simulink model "sim_tase_2025_pos_ctrl"  (R2020a)
settings: Solver=ode4  StartTime=0.0  StopTime=30.0  FixedStep=0.01  RelTol=1e-3
values from neighbouring files (symbols this model uses):
  alfa_theta_obs = 100    [init_tase_2025_pos_ctrl.m]
  Aps = -diag([5, 5, 5])    [init_tase_2025_pos_ctrl.m]
  delta_p_i_0 = zeros(3, NF)    [init_tase_2025_pos_ctrl.m]
  delta_v_i_0 = zeros(3, NF)    [init_tase_2025_pos_ctrl.m]
  dp_aa_t = 0.2 * ones(3, 5) + ( 1.0 - 0.2 ) * rand(3, 5)    [init_tase_2025_pos_ctrl.m]
  dp_ff_t = [ 0.4 * ones(1, 5) + ( 1.0 - 0.4 ) * rand(1, 5);                      0.4 * ones(1, 5) + ( 1.0 - 0.4 ) * rand(1, 5);                      0.2 * ones(1, 5) + ( 0.6 - 0.2 ) * rand(1, 5) ]    [init_tase_2025_pos_ctrl.m]
  dp_phi_t = ( - pi / 2 ) * ones(3, 5) + ( pi / 2 - ( - pi / 2 ) ) * rand(3, 5)    [init_tase_2025_pos_ctrl.m]
  etai_0 = zeros(3,5)    [init_tase_2025_pos_ctrl.m]
  k_rho_1 = 10    [init_tase_2025_pos_ctrl.m]
  k_rho_2 = 10    [init_tase_2025_pos_ctrl.m]
  kai_1_t = 0.02    [init_tase_2025_pos_ctrl.m]
  kai_3_t = 0.1    [init_tase_2025_pos_ctrl.m]
  kp = 20    [init_tase_2025_pos_ctrl.m]
  ksii_0 = zeros(3,5)    [init_tase_2025_pos_ctrl.m]
  kv = 20    [init_tase_2025_pos_ctrl.m]
  l1v = diag([20; 20; 20])    [init_tase_2025_pos_ctrl.m]
  l2v = diag([30; 30; 30])    [init_tase_2025_pos_ctrl.m]
  mass_i = zeros(1,NF)    [init_tase_2025_pos_ctrl.m]
  Mii = diag([1;0;0;0;1])    [init_tase_2025_pos_ctrl.m]
  Phi_inv = inv( Aps ) * ( exp( Aps * tTs ) - eye(3) )    [init_tase_2025_pos_ctrl.m]
  pos0 = zeros(3, 1)    [init_tase_2025_pos_ctrl.m]
  PZ0 = P0(3)    [init_tase_2025_pos_ctrl.m]
  PZ1 = 10    [init_tase_2025_pos_ctrl.m]
  Qci_init = repmat([1;0;0;0],1,NF)    [init_tase_2025_pos_ctrl.m]
  R0 = 4    [init_tase_2025_pos_ctrl.m]
  R1 = 8    [init_tase_2025_pos_ctrl.m]
  Rx2 = 10    [init_tase_2025_pos_ctrl.m]
  Ry2 = 6    [init_tase_2025_pos_ctrl.m]
  Rz2 = 4    [init_tase_2025_pos_ctrl.m]
  T0 = 0    [init_tase_2025_pos_ctrl.m]
  T1 = tseq1    (= 10)    [init_tase_2025_pos_ctrl.m]
  T12 = tseq1 + tseq12    (= 20)    [init_tase_2025_pos_ctrl.m]
  T2 = tseq1 + tseq12 + tseq2    (= 30)    [init_tase_2025_pos_ctrl.m]
  theta0 = ( 2 / 5 ) * pi    (= 1.25663706144)    [init_tase_2025_pos_ctrl.m]
  theta_1 = 0    [init_tase_2025_pos_ctrl.m]
  theta_2 = 1    [init_tase_2025_pos_ctrl.m]
  TTb = 2    [init_tase_2025_pos_ctrl.m]
  tTs = 0.1    [init_tase_2025_pos_ctrl.m]
  vel0 = zeros(3, 1)    [init_tase_2025_pos_ctrl.m]
  Wij = [0,0,1,0,0;              0,0,1,1,0;              1,0,0,0,1;              0,1,1,0,0;              0,0,1,0,0]    [init_tase_2025_pos_ctrl.m]
  wp = 10    [init_tase_2025_pos_ctrl.m]
  X1 = 8    [init_tase_2025_pos_ctrl.m]
  X2 = 2    [init_tase_2025_pos_ctrl.m]
  X3 = 3    [init_tase_2025_pos_ctrl.m]
  Y1 = 10    [init_tase_2025_pos_ctrl.m]
  Y2 = 2    [init_tase_2025_pos_ctrl.m]
  Y3 = 4    [init_tase_2025_pos_ctrl.m]
  Z1 = 4    [init_tase_2025_pos_ctrl.m]
  Z2 = -6    [init_tase_2025_pos_ctrl.m]
  Z3 = 2    [init_tase_2025_pos_ctrl.m]
undefined symbols (not defined in the file or in its folder): cal_frac_squ, p_gamma1_pos, p_gamma1_vel, p_gamma2_pos, p_gamma2_vel, p_gamma_diff_1, p_gamma_diff_2_2, q_gamma1_pos, q_gamma1_vel, q_gamma2_pos, q_gamma2_vel, q_gamma_diff_1, q_gamma_diff_2_2
(part 3 of 4)

== matlab function sim_tase_2025_pos_ctrl/combine leader position estimaters ==
  data: ksi_d_est_1 input; ksi_d_est_vec output; ksi_d_est_2 input; ksi_d_est_3 input; ksi_d_est_4 input; ksi_d_est_5 input
function ksi_d_est_vec  = fcn(ksi_d_est_1, ksi_d_est_2, ksi_d_est_3, ksi_d_est_4, ksi_d_est_5)
%%%% 合并领导者位置观测器输出结果
ksi_d_est_vec = [ksi_d_est_1(:), ksi_d_est_2(:), ksi_d_est_3(:), ksi_d_est_4(:), ksi_d_est_5(:)];

== matlab function sim_tase_2025_pos_ctrl/combine lumped follower observation error  ==
  data: ksi_est_err_tilt_1 input; ksi_est_err_tilt_2 input; ksi_est_err_tilt_3 input; ksi_est_err_tilt_4 input; ksi_est_err_tilt_5 input; ksi_est_err_tilt_vec output; eta_est_err_tilt_1 input; eta_est_err_tilt_vec output; eta_est_err_tilt_2 input; eta_est_err_tilt_3 input; eta_est_err_tilt_4 input; eta_est_err_tilt_5 input
function [ksi_est_err_tilt_vec, eta_est_err_tilt_vec]  = fcn(ksi_est_err_tilt_1, ksi_est_err_tilt_2, ksi_est_err_tilt_3, ksi_est_err_tilt_4, ksi_est_err_tilt_5, ...
                                                                                                        eta_est_err_tilt_1, eta_est_err_tilt_2, eta_est_err_tilt_3, eta_est_err_tilt_4, eta_est_err_tilt_5)
%%%% 合并领导者位置观测器输出结果
ksi_est_err_tilt_vec = [ksi_est_err_tilt_1, ksi_est_err_tilt_2, ksi_est_err_tilt_3, ksi_est_err_tilt_4, ksi_est_err_tilt_5];
eta_est_err_tilt_vec = [eta_est_err_tilt_1, eta_est_err_tilt_2, eta_est_err_tilt_3, eta_est_err_tilt_4, eta_est_err_tilt_5];

== matlab function sim_tase_2025_pos_ctrl/combine lumped follower position observation error ==
  data: theta_ksi_est_err_tilt_1_1 input; theta_ksi_est_err_tilt_1_2 input; theta_ksi_est_err_tilt_1_3 input; theta_ksi_est_err_tilt_1_4 input; theta_ksi_est_err_tilt_1_5 input; theta_ksi_est_err_tilt_1_vec output; theta_ksi_est_err_tilt_2_1 input; theta_ksi_est_err_tilt_2_vec output; theta_ksi_est_err_tilt_2_2 input; theta_ksi_est_err_tilt_2_3 input; theta_ksi_est_err_tilt_2_4 input; theta_ksi_est_err_tilt_2_5 input
function [theta_ksi_est_err_tilt_1_vec, theta_ksi_est_err_tilt_2_vec]  = fcn(theta_ksi_est_err_tilt_1_1, theta_ksi_est_err_tilt_1_2, theta_ksi_est_err_tilt_1_3, theta_ksi_est_err_tilt_1_4, theta_ksi_est_err_tilt_1_5, ...
                                                                                                                                    theta_ksi_est_err_tilt_2_1, theta_ksi_est_err_tilt_2_2, theta_ksi_est_err_tilt_2_3, theta_ksi_est_err_tilt_2_4, theta_ksi_est_err_tilt_2_5)
%%%% 合并领导者位置观测器输出结果
theta_ksi_est_err_tilt_1_vec = [theta_ksi_est_err_tilt_1_1(:), theta_ksi_est_err_tilt_1_2(:), theta_ksi_est_err_tilt_1_3(:), theta_ksi_est_err_tilt_1_4(:), theta_ksi_est_err_tilt_1_5(:)];
theta_ksi_est_err_tilt_2_vec = [theta_ksi_est_err_tilt_2_1(:), theta_ksi_est_err_tilt_2_2(:), theta_ksi_est_err_tilt_2_3(:), theta_ksi_est_err_tilt_2_4(:), theta_ksi_est_err_tilt_2_5(:)];

== matlab function sim_tase_2025_pos_ctrl/combine lumped follower velocity observation error ==
  data: theta_eta_est_err_tilt_1_1 input; theta_eta_est_err_tilt_1_2 input; theta_eta_est_err_tilt_1_3 input; theta_eta_est_err_tilt_1_4 input; theta_eta_est_err_tilt_1_5 input; theta_eta_est_err_tilt_1_vec output; theta_eta_est_err_tilt_2_1 input; theta_eta_est_err_tilt_2_vec output; theta_eta_est_err_tilt_2_2 input; theta_eta_est_err_tilt_2_3 input; theta_eta_est_err_tilt_2_4 input; theta_eta_est_err_tilt_2_5 input
function [theta_eta_est_err_tilt_1_vec, theta_eta_est_err_tilt_2_vec]  = fcn(theta_eta_est_err_tilt_1_1, theta_eta_est_err_tilt_1_2, theta_eta_est_err_tilt_1_3, theta_eta_est_err_tilt_1_4, theta_eta_est_err_tilt_1_5, ...
                                                                                                                                    theta_eta_est_err_tilt_2_1, theta_eta_est_err_tilt_2_2, theta_eta_est_err_tilt_2_3, theta_eta_est_err_tilt_2_4, theta_eta_est_err_tilt_2_5)
%%%% 合并领导者位置观测器输出结果
theta_eta_est_err_tilt_1_vec = [theta_eta_est_err_tilt_1_1(:), theta_eta_est_err_tilt_1_2(:), theta_eta_est_err_tilt_1_3(:), theta_eta_est_err_tilt_1_4(:), theta_eta_est_err_tilt_1_5(:)];
theta_eta_est_err_tilt_2_vec = [theta_eta_est_err_tilt_2_1(:), theta_eta_est_err_tilt_2_2(:), theta_eta_est_err_tilt_2_3(:), theta_eta_est_err_tilt_2_4(:), theta_eta_est_err_tilt_2_5(:)];

== matlab function sim_tase_2025_pos_ctrl/fixed-time distributed follower desire position observer agent 1 ==
  data: l1p input; d_ksi_d_est_1 output; l2p input; eta_d_est_vec input; theta_ksi_est_err_tilt_1_vec input; theta_ksi_est_err_tilt_2_vec input
function d_ksi_d_est_1 = fcn(l1p, l2p, eta_d_est_vec, theta_ksi_est_err_tilt_1_vec, theta_ksi_est_err_tilt_2_vec)
%%%% 固定时间跟随者期望位置分布式观测器
iiuav = 1;
d_ksi_d_est_1 = eta_d_est_vec(:,iiuav) - l1p * theta_ksi_est_err_tilt_1_vec(:,iiuav) - l2p * theta_ksi_est_err_tilt_2_vec(:,iiuav);

== matlab function sim_tase_2025_pos_ctrl/fixed-time distributed follower desire position observer agent 2 ==
  data: l1p input; d_ksi_d_est_2 output; l2p input; eta_d_est_vec input; theta_ksi_est_err_tilt_1_vec input; theta_ksi_est_err_tilt_2_vec input
function d_ksi_d_est_2 = fcn(l1p, l2p, eta_d_est_vec, theta_ksi_est_err_tilt_1_vec, theta_ksi_est_err_tilt_2_vec)
%%%% 固定时间跟随者期望位置分布式观测器
iiuav = 2;
d_ksi_d_est_2 = eta_d_est_vec(:,iiuav) - l1p * theta_ksi_est_err_tilt_1_vec(:,iiuav) - l2p * theta_ksi_est_err_tilt_2_vec(:,iiuav);

== matlab function sim_tase_2025_pos_ctrl/update vl_hat agent 2 ==
  data: Aps input; d_vl_hat_2 output; ui0 input; ui1 input; dp_hat_vec input; vli_tilt_vec input
function d_vl_hat_2 = fcn(Aps, ui0, ui1, dp_hat_vec, vli_tilt_vec)
%%%% 更新状态预测器
iiuav = 2;
g0 = 9.80663;
e3 = [0;0;1];
d_vl_hat_2 = -g0 * e3 + ui0(:,iiuav) + dp_hat_vec(:,iiuav) ...
                        + ui1(:,iiuav) + Aps * vli_tilt_vec(:,iiuav);

== matlab function sim_tase_2025_pos_ctrl/fixed-time distributed follower desire position observer agent 3 ==
  data: l1p input; d_ksi_d_est_3 output; l2p input; eta_d_est_vec input; theta_ksi_est_err_tilt_1_vec input; theta_ksi_est_err_tilt_2_vec input
function d_ksi_d_est_3 = fcn(l1p, l2p, eta_d_est_vec, theta_ksi_est_err_tilt_1_vec, theta_ksi_est_err_tilt_2_vec)
%%%% 固定时间跟随者期望位置分布式观测器
iiuav = 3;
d_ksi_d_est_3 = eta_d_est_vec(:,iiuav) - l1p * theta_ksi_est_err_tilt_1_vec(:,iiuav) - l2p * theta_ksi_est_err_tilt_2_vec(:,iiuav);

== matlab function sim_tase_2025_pos_ctrl/fixed-time distributed follower desire position observer agent 4 ==
  data: l1p input; d_ksi_d_est_4 output; l2p input; eta_d_est_vec input; theta_ksi_est_err_tilt_1_vec input; theta_ksi_est_err_tilt_2_vec input
function d_ksi_d_est_4 = fcn(l1p, l2p, eta_d_est_vec, theta_ksi_est_err_tilt_1_vec, theta_ksi_est_err_tilt_2_vec)
%%%% 固定时间跟随者期望位置分布式观测器
iiuav = 4;
d_ksi_d_est_4 = eta_d_est_vec(:,iiuav) - l1p * theta_ksi_est_err_tilt_1_vec(:,iiuav) - l2p * theta_ksi_est_err_tilt_2_vec(:,iiuav);

== matlab function sim_tase_2025_pos_ctrl/fixed-time distributed follower desire position observer agent 5 ==
  data: l1p input; d_ksi_d_est_5 output; l2p input; eta_d_est_vec input; theta_ksi_est_err_tilt_1_vec input; theta_ksi_est_err_tilt_2_vec input
function d_ksi_d_est_5 = fcn(l1p, l2p, eta_d_est_vec, theta_ksi_est_err_tilt_1_vec, theta_ksi_est_err_tilt_2_vec)
%%%% 固定时间跟随者期望位置分布式观测器
iiuav = 5;
d_ksi_d_est_5 = eta_d_est_vec(:,iiuav) - l1p * theta_ksi_est_err_tilt_1_vec(:,iiuav) - l2p * theta_ksi_est_err_tilt_2_vec(:,iiuav);

== matlab function sim_tase_2025_pos_ctrl/fixed-time distributed follower desire velocity observer agent 1 ==
  data: l1v input; d_eta_d_est_1 output; l2v input; theta_eta_est_err_tilt_1_vec input; theta_eta_est_err_tilt_2_vec input
function d_eta_d_est_1 = fcn(l1v, l2v, theta_eta_est_err_tilt_1_vec, theta_eta_est_err_tilt_2_vec)
%%%% 固定时间跟随者期望速度分布式观测器
iiuav = 1;
d_eta_d_est_1 = -l1v * theta_eta_est_err_tilt_1_vec(:,iiuav) - l2v * theta_eta_est_err_tilt_2_vec(:,iiuav);

== matlab function sim_tase_2025_pos_ctrl/fixed-time distributed follower desire velocity observer agent 2 ==
  data: l1v input; d_eta_d_est_2 output; l2v input; theta_eta_est_err_tilt_1_vec input; theta_eta_est_err_tilt_2_vec input
function d_eta_d_est_2 = fcn(l1v, l2v, theta_eta_est_err_tilt_1_vec, theta_eta_est_err_tilt_2_vec)
%%%% 固定时间跟随者期望速度分布式观测器
iiuav = 2;
d_eta_d_est_2 = -l1v * theta_eta_est_err_tilt_1_vec(:,iiuav) - l2v * theta_eta_est_err_tilt_2_vec(:,iiuav);

== matlab function sim_tase_2025_pos_ctrl/fixed-time distributed follower desire velocity observer agent 3 ==
  data: l1v input; d_eta_d_est_3 output; l2v input; theta_eta_est_err_tilt_1_vec input; theta_eta_est_err_tilt_2_vec input
function d_eta_d_est_3 = fcn(l1v, l2v, theta_eta_est_err_tilt_1_vec, theta_eta_est_err_tilt_2_vec)
%%%% 固定时间跟随者期望速度分布式观测器
iiuav = 3;
d_eta_d_est_3 = -l1v * theta_eta_est_err_tilt_1_vec(:,iiuav) - l2v * theta_eta_est_err_tilt_2_vec(:,iiuav);

== matlab function sim_tase_2025_pos_ctrl/fixed-time distributed follower desire velocity observer agent 4 ==
  data: l1v input; d_eta_d_est_4 output; l2v input; theta_eta_est_err_tilt_1_vec input; theta_eta_est_err_tilt_2_vec input
function d_eta_d_est_4 = fcn(l1v, l2v, theta_eta_est_err_tilt_1_vec, theta_eta_est_err_tilt_2_vec)
%%%% 固定时间跟随者期望速度分布式观测器
iiuav = 4;
d_eta_d_est_4 = -l1v * theta_eta_est_err_tilt_1_vec(:,iiuav) - l2v * theta_eta_est_err_tilt_2_vec(:,iiuav);

== matlab function sim_tase_2025_pos_ctrl/fixed-time distributed follower desire velocity observer agent 5 ==
  data: l1v input; d_eta_d_est_5 output; l2v input; theta_eta_est_err_tilt_1_vec input; theta_eta_est_err_tilt_2_vec input
function d_eta_d_est_5 = fcn(l1v, l2v, theta_eta_est_err_tilt_1_vec, theta_eta_est_err_tilt_2_vec)
%%%% 固定时间跟随者期望速度分布式观测器
iiuav = 5;
d_eta_d_est_5 = -l1v * theta_eta_est_err_tilt_1_vec(:,iiuav) - l2v * theta_eta_est_err_tilt_2_vec(:,iiuav);

== matlab function sim_tase_2025_pos_ctrl/trans to column41 ==
  data: x input; y output
function y = fcn(x)
y = x(:);

== matlab function sim_tase_2025_pos_ctrl/trans to column42 ==
  data: x input; y output
function y = fcn(x)
y = x(:);

== matlab function sim_tase_2025_pos_ctrl/trans to column43 ==
  data: x input; y output
function y = fcn(x)
y = x(:);

== matlab function sim_tase_2025_pos_ctrl/update vl_hat agent 3 ==
  data: Aps input; d_vl_hat_3 output; ui0 input; ui1 input; dp_hat_vec input; vli_tilt_vec input
function d_vl_hat_3 = fcn(Aps, ui0, ui1, dp_hat_vec, vli_tilt_vec)
%%%% 更新状态预测器
iiuav = 3;
g0 = 9.80663;
e3 = [0;0;1];
d_vl_hat_3 = -g0 * e3 + ui0(:,iiuav) + dp_hat_vec(:,iiuav) ...
                        + ui1(:,iiuav) + Aps * vli_tilt_vec(:,iiuav);

== matlab function sim_tase_2025_pos_ctrl/trans to column44 ==
  data: x input; y output
function y = fcn(x)
y = x(:);

== matlab function sim_tase_2025_pos_ctrl/trans to column45 ==
  data: x input; y output
function y = fcn(x)
y = x(:);

== matlab function sim_tase_2025_pos_ctrl/trans to column46 ==
  data: x input; y output
function y = fcn(x)
y = x(:);

== matlab function sim_tase_2025_pos_ctrl/trans to column47 ==
  data: x input; y output
function y = fcn(x)
y = x(:);

== matlab function sim_tase_2025_pos_ctrl/trans to column48 ==
  data: x input; y output
function y = fcn(x)
y = x(:);

== matlab function sim_tase_2025_pos_ctrl/trans to column49 ==
  data: x input; y output
function y = fcn(x)
y = x(:);

== matlab function sim_tase_2025_pos_ctrl/trans to column50 ==
  data: x input; y output
function y = fcn(x)
y = x(:);

== matlab function sim_tase_2025_pos_ctrl/trans to column51 ==
  data: x input; y output
function y = fcn(x)
y = x(:);

== matlab function sim_tase_2025_pos_ctrl/trans to column52 ==
  data: x input; y output
function y = fcn(x)
y = x(:);

== matlab function sim_tase_2025_pos_ctrl/trans to column53 ==
  data: x input; y output
function y = fcn(x)
y = x(:);

== matlab function sim_tase_2025_pos_ctrl/trans to column54 ==
  data: x input; y output
function y = fcn(x)
y = x(:);

== matlab function sim_tase_2025_pos_ctrl/trans to column55 ==
  data: x input; y output
function y = fcn(x)
y = x(:);

== matlab function sim_tase_2025_pos_ctrl/trans to column56 ==
  data: x input; y output
function y = fcn(x)
y = x(:);

== matlab function sim_tase_2025_pos_ctrl/trans to column57 ==
  data: x input; y output
function y = fcn(x)
y = x(:);

== matlab function sim_tase_2025_pos_ctrl/trans to column58 ==
  data: x input; y output
function y = fcn(x)
y = x(:);

== matlab function sim_tase_2025_pos_ctrl/trans to column59 ==
  data: x input; y output
function y = fcn(x)
y = x(:);

== matlab function sim_tase_2025_pos_ctrl/update vl_hat agent 4 ==
  data: Aps input; d_vl_hat_4 output; ui0 input; ui1 input; dp_hat_vec input; vli_tilt_vec input
function d_vl_hat_4 = fcn(Aps, ui0, ui1, dp_hat_vec, vli_tilt_vec)
%%%% 更新状态预测器
iiuav = 4;
g0 = 9.80663;
e3 = [0;0;1];
d_vl_hat_4 = -g0 * e3 + ui0(:,iiuav) + dp_hat_vec(:,iiuav) ...
                        + ui1(:,iiuav) + Aps * vli_tilt_vec(:,iiuav);

== matlab function sim_tase_2025_pos_ctrl/trans to column60 ==
  data: x input; y output
function y = fcn(x)
y = x(:);

== matlab function sim_tase_2025_pos_ctrl/update vl_hat agent 5 ==
  data: Aps input; d_vl_hat_5 output; ui0 input; ui1 input; dp_hat_vec input; vli_tilt_vec input
function d_vl_hat_5 = fcn(Aps, ui0, ui1, dp_hat_vec, vli_tilt_vec)
%%%% 更新状态预测器
iiuav = 5;
g0 = 9.80663;
e3 = [0;0;1];
d_vl_hat_5 = -g0 * e3 + ui0(:,iiuav) + dp_hat_vec(:,iiuav) ...
                        + ui1(:,iiuav) + Aps * vli_tilt_vec(:,iiuav);

== matlab function sim_tase_2025_pos_ctrl/combine vl_hat ==
  data: vl_hat_1 input; vl_hat_2 input; vl_hat_3 input; vl_hat_4 input; vl_hat_5 input; vl_hat_vec output
function vl_hat_vec  = fcn(vl_hat_1, vl_hat_2, vl_hat_3, vl_hat_4, vl_hat_5)
%%%% 合并速度预测器
vl_hat_vec = [vl_hat_1(:), vl_hat_2(:), vl_hat_3(:), vl_hat_4(:), vl_hat_5(:)];

== matlab function sim_tase_2025_pos_ctrl/cal vl_tilt prediction error ==
  data: eta_i_vec input; vl_tilt_vec output; vl_hat_vec input
function vl_tilt_vec = fcn(eta_i_vec, vl_hat_vec)
%%%% 计算速度预测误差
vl_tilt_vec = zeros(3,5);
for iiuav = 1:5
    vl_tilt_vec(:,iiuav) = vl_hat_vec(:,iiuav) - eta_i_vec(:,iiuav);
end

== matlab function sim_tase_2025_pos_ctrl/cal sample vl_tilt ==
  data: tTs input; vl_tilt_bTs_vec output; tsim input; vl_tilt_vec input; vl_tilt_bTs_vec input
function vl_tilt_bTs_vec = fcn(tTs, tsim, vl_tilt_vec, vl_tilt_bTs_vec)
%%%% 对速度预测误差进行采样
nn = fix( tsim / tTs );
if abs( nn - ( tsim / tTs ) ) <= 1e-04
    for iiuav = 1:5
        vl_tilt_bTs_vec(:,iiuav) = vl_tilt_vec(:,iiuav);
    end
end

== matlab function sim_tase_2025_pos_ctrl/cal mu_bTs_vec ==
  data: mu_bTs_vec output; Aps input; vl_tilt_bTs_vec input
function mu_bTs_vec = fcn(Aps, vl_tilt_bTs_vec)
%%%% 计算扰动观测器辅助误差向量
mu_bTs_vec = zeros(3,5);
for iiuav = 1:5
    mu_bTs_vec(:,iiuav) = exp( Aps ) * vl_tilt_bTs_vec(:,iiuav);
end

== matlab function sim_tase_2025_pos_ctrl/cal dp_hat agent 2 ==
  data: Phi_inv input; mu_bTs_vec input; dp_hat_2 output
function dp_hat_2 = fcn(Phi_inv, mu_bTs_vec)
%%%% 计算扰动观测值dp_hat
iiuav = 2;
dp_hat_2 = -Phi_inv * mu_bTs_vec(:,iiuav);

== matlab function sim_tase_2025_pos_ctrl/cal position and velocity signal tracking errors ==
  data: ksi_i_vec input; err_ksi_vec output; ksi_d_est_vec input; eta_i_vec input; eta_d_est_vec input; err_eta_vec output
function [err_ksi_vec, err_eta_vec] = fcn(ksi_i_vec, ksi_d_est_vec, eta_i_vec, eta_d_est_vec)
%%%% 计算编队跟踪误差
err_ksi_vec = zeros(3,5);
err_eta_vec = zeros(3,5);
for iiuav = 1:5
    err_ksi_vec(:,iiuav) = ksi_i_vec(:,iiuav) - ksi_d_est_vec(:,iiuav);
    err_eta_vec(:,iiuav) = eta_i_vec(:,iiuav) - eta_d_est_vec(:,iiuav);
end

== matlab function sim_tase_2025_pos_ctrl/cal dp_hat agent 3 ==
  data: Phi_inv input; mu_bTs_vec input; dp_hat_3 output
function dp_hat_3 = fcn(Phi_inv, mu_bTs_vec)
%%%% 计算扰动观测值dp_hat
iiuav = 3;
dp_hat_3 = -Phi_inv * mu_bTs_vec(:,iiuav);

== matlab function sim_tase_2025_pos_ctrl/cal dp_hat agent 4 ==
  data: Phi_inv input; mu_bTs_vec input; dp_hat_4 output
function dp_hat_4 = fcn(Phi_inv, mu_bTs_vec)
%%%% 计算扰动观测值dp_hat
iiuav = 4;
dp_hat_4 = -Phi_inv * mu_bTs_vec(:,iiuav);

== matlab function sim_tase_2025_pos_ctrl/cal dp_hat agent 5 ==
  data: Phi_inv input; mu_bTs_vec input; dp_hat_5 output
function dp_hat_5 = fcn(Phi_inv, mu_bTs_vec)
%%%% 计算扰动观测值dp_hat
iiuav = 5;
dp_hat_5 = -Phi_inv * mu_bTs_vec(:,iiuav);

== matlab function sim_tase_2025_pos_ctrl/choose dp_hat agent 1 ==
  data: x input; y output
function y = fcn(x)
iiuav = 1;
y = x(:,iiuav);

== matlab function sim_tase_2025_pos_ctrl/choose dp_hat agent 2 ==
  data: x input; y output
function y = fcn(x)
iiuav = 2;
y = x(:,iiuav);

== matlab function sim_tase_2025_pos_ctrl/choose dp_hat agent 3 ==
  data: x input; y output
function y = fcn(x)
iiuav = 3;
y = x(:,iiuav);

== matlab function sim_tase_2025_pos_ctrl/choose dp_hat agent 4 ==
  data: x input; y output
function y = fcn(x)
iiuav = 4;
y = x(:,iiuav);

== matlab function sim_tase_2025_pos_ctrl/choose dp_hat agent 5 ==
  data: x input; y output
function y = fcn(x)
iiuav = 5;
y = x(:,iiuav);

== matlab function sim_tase_2025_pos_ctrl/combine ui1_vec ==
  data: ui1_1 input; ui1_2 input; ui1_3 input; ui1_4 input; ui1_5 input; ui1 output
function ui1  = fcn(ui1_1, ui1_2, ui1_3, ui1_4, ui1_5)
%%%% 合并控制输入补偿项
ui1 = [ui1_1(:), ui1_2(:), ui1_3(:), ui1_4(:), ui1_5(:)];

== matlab function sim_tase_2025_pos_ctrl/cal control input ui ==
  data: ui0 input; ui output; ui1 input
function ui = fcn(ui0, ui1)
ui = zeros(3,5);
for iiuav = 1:5
    ui(:,iiuav) = ui0(:,iiuav) + ui1(:,iiuav);
end

== matlab function sim_tase_2025_pos_ctrl/cal high-order sliding mode differentiator position estimation error ==
  data: ksi_i_vec input; ksi_diff_tilt_vec output; pos_diff_hat_vec input
function ksi_diff_tilt_vec = fcn(ksi_i_vec, pos_diff_hat_vec)
%%%% 计算高阶滑模微分器的位置状态估计误差
ksi_diff_tilt_vec = zeros(3,5);
for iiuav = 1:5
    ksi_diff_tilt_vec(:,iiuav) = pos_diff_hat_vec(:,iiuav) - ksi_i_vec(:,iiuav);
end

== matlab function sim_tase_2025_pos_ctrl/combine formation control input ==
  data: eta_i_vec output; ksi_i_vec output; eta_1 input; eta_2 input; eta_3 input; eta_4 input; eta_5 input; ksi_1 input; ksi_2 input; ksi_3 input; ksi_4 input; ksi_5 input
function [eta_i_vec, ksi_i_vec] = fcn(eta_1, eta_2, eta_3, eta_4, eta_5, ...
                                                                ksi_1, ksi_2, ksi_3, ksi_4, ksi_5)
%%%% 合并领导者编队跟踪误差结果
eta_i_vec = [eta_1(:), eta_2(:), eta_3(:), eta_4(:), eta_5(:)];
ksi_i_vec = [ksi_1(:), ksi_2(:), ksi_3(:), ksi_4(:), ksi_5(:)];

== matlab function sim_tase_2025_pos_ctrl/cal vel_diff_hat agent 1 ==
  data: k_rho_1 input; k_rho_2 input; TTb input; theta_1 input; theta_2 input; tsim input; ksi_diff_tilt_vec input; d_vel_diff_hat_1 output; sig_ksi_diff_tilt_gamma_1_vec input
function d_vel_diff_hat_1 = fcn(k_rho_1, k_rho_2, TTb, theta_1, theta_2, tsim, ksi_diff_tilt_vec, sig_ksi_diff_tilt_gamma_1_vec)
%%%% 计算高阶滑模微分器的速度估计
iiuav = 1;
if tsim < TTb
    theta = theta_1;
else
    theta = theta_2;
end
d_vel_diff_hat_1 = -theta * k_rho_1 * sign( ksi_diff_tilt_vec(:,iiuav) ) ...
                                    - ( 1 - theta ) * k_rho_2 * sig_ksi_diff_tilt_gamma_1_vec(:,iiuav);

== matlab function sim_tase_2025_pos_ctrl/cal abs 1 ==
  data: x input; y output
function y = fcn(x)
y = abs(x(:));

== matlab function sim_tase_2025_pos_ctrl/choose ksi_diff_tilt 2 ==
  data: x input; y output
function y = fcn(x)
iiuav = 1;
y = x(:,iiuav);

== matlab function sim_tase_2025_pos_ctrl/trans to column1 ==
  data: x input; y output
function y = fcn(x)
y = x(:);

== matlab function sim_tase_2025_pos_ctrl/uav translational dynamics agent 1 ==
  data: dvi output; Ri input; ui input; dpi_vec input
function dvi = fcn(Ri, ui, dpi_vec)
%%%% 根据有限时间控制输入计算无人机平移动力学微分方程
iiuav = 1;
g0 = 9.80663;
e3 = [0;0;1];
dvi = -g0 * e3 + norm(ui(:,iiuav),2) * Ri(:,:,iiuav) * e3 + dpi_vec(:,iiuav);

== matlab function sim_tase_2025_pos_ctrl/uav translational dynamics agent 2 ==
  data: dvi output; Ri input; ui input; dpi_vec input
function dvi = fcn(Ri, ui, dpi_vec)
%%%% 根据有限时间控制输入计算无人机平移动力学微分方程
iiuav = 2;
g0 = 9.80663;
e3 = [0;0;1];
dvi = -g0 * e3 + norm(ui(:,iiuav),2) * Ri(:,:,iiuav) * e3 + dpi_vec(:,iiuav);

== matlab function sim_tase_2025_pos_ctrl/uav translational dynamics agent 3 ==
  data: dvi output; Ri input; ui input; dpi_vec input
function dvi = fcn(Ri, ui, dpi_vec)
%%%% 根据有限时间控制输入计算无人机平移动力学微分方程
iiuav = 3;
g0 = 9.80663;
e3 = [0;0;1];
dvi = -g0 * e3 + norm(ui(:,iiuav),2) * Ri(:,:,iiuav) * e3 + dpi_vec(:,iiuav);

== matlab function sim_tase_2025_pos_ctrl/uav translational dynamics agent 4 ==
  data: dvi output; Ri input; ui input; dpi_vec input
function dvi = fcn(Ri, ui, dpi_vec)
%%%% 根据有限时间控制输入计算无人机平移动力学微分方程
iiuav = 4;
g0 = 9.80663;
e3 = [0;0;1];
dvi = -g0 * e3 + norm(ui(:,iiuav),2) * Ri(:,:,iiuav) * e3 + dpi_vec(:,iiuav);

== matlab function sim_tase_2025_pos_ctrl/uav translational dynamics agent 5 ==
  data: dvi output; Ri input; ui input; dpi_vec input
function dvi = fcn(Ri, ui, dpi_vec)
%%%% 根据有限时间控制输入计算无人机平移动力学微分方程
iiuav = 5;
g0 = 9.80663;
e3 = [0;0;1];
dvi = -g0 * e3 + norm(ui(:,iiuav),2) * Ri(:,:,iiuav) * e3 + dpi_vec(:,iiuav);

== matlab function sim_tase_2025_pos_ctrl/cal Ri ==
  data: Ri output; Rei input; Rci input
function Ri = fcn(Rei, Rci)
%%%% 使用罗德里格公式由四元数Qci求解Rci
Ri = zeros(3,3,5);
for iiuav = 1:5
    Ri(:,:,iiuav) = Rci(:,:,iiuav) * Rei(:,:,iiuav);
end

end

== matlab function sim_tase_2025_pos_ctrl/follower tracking error agent 1 ==
  data: ksi_track_err_1 output; delta_ksi_vec input; delta_eta_vec input; ksi_i_vec input; eta_i_vec input; ksi0 input; eta_track_err_1 output; eta0 input
function [ksi_track_err_1, eta_track_err_1]  = fcn(delta_ksi_vec, delta_eta_vec, ksi_i_vec, eta_i_vec, ksi0, eta0)
%%%% 计算跟随者节点1号位置/速度跟踪误差
eta_track_err_1 = eta_i_vec(:,1) - delta_eta_vec(:,1) - eta0;
ksi_track_err_1 = ksi_i_vec(:,1) - delta_ksi_vec(:,1) - ksi0;

== matlab function sim_tase_2025_pos_ctrl/follower tracking error agent 2 ==
  data: ksi_track_err_2 output; delta_ksi_vec input; delta_eta_vec input; ksi_i_vec input; eta_i_vec input; ksi0 input; eta_track_err_2 output; eta0 input
function [ksi_track_err_2, eta_track_err_2]  = fcn(delta_ksi_vec, delta_eta_vec, ksi_i_vec, eta_i_vec, ksi0, eta0)
%%%% 计算跟随者节点2号位置/速度跟踪误差
eta_track_err_2 = eta_i_vec(:,2) - delta_eta_vec(:,2) - eta0;
ksi_track_err_2 = ksi_i_vec(:,2) - delta_ksi_vec(:,2) - ksi0;

== matlab function sim_tase_2025_pos_ctrl/follower tracking error agent 3 ==
  data: ksi_track_err_3 output; delta_ksi_vec input; delta_eta_vec input; ksi_i_vec input; eta_i_vec input; ksi0 input; eta_track_err_3 output; eta0 input
function [ksi_track_err_3, eta_track_err_3]  = fcn(delta_ksi_vec, delta_eta_vec, ksi_i_vec, eta_i_vec, ksi0, eta0)
%%%% 计算跟随者节点3号位置/速度跟踪误差
eta_track_err_3 = eta_i_vec(:,3) - delta_eta_vec(:,3) - eta0;
ksi_track_err_3 = ksi_i_vec(:,3) - delta_ksi_vec(:,3) - ksi0;

== matlab function sim_tase_2025_pos_ctrl/follower tracking error agent 4 ==
  data: ksi_track_err_4 output; delta_ksi_vec input; delta_eta_vec input; ksi_i_vec input; eta_i_vec input; ksi0 input; eta_track_err_4 output; eta0 input
function [ksi_track_err_4, eta_track_err_4]  = fcn(delta_ksi_vec, delta_eta_vec, ksi_i_vec, eta_i_vec, ksi0, eta0)
%%%% 计算跟随者节点4号位置/速度跟踪误差
eta_track_err_4 = eta_i_vec(:,4) - delta_eta_vec(:,4) - eta0;
ksi_track_err_4 = ksi_i_vec(:,4) - delta_ksi_vec(:,4) - ksi0;

== matlab function sim_tase_2025_pos_ctrl/follower tracking error agent 5 ==
  data: ksi_track_err_5 output; delta_ksi_vec input; delta_eta_vec input; ksi_i_vec input; eta_i_vec input; ksi0 input; eta_track_err_5 output; eta0 input
function [ksi_track_err_5, eta_track_err_5]  = fcn(delta_ksi_vec, delta_eta_vec, ksi_i_vec, eta_i_vec, ksi0, eta0)
%%%% 计算跟随者节点5号位置/速度跟踪误差
eta_track_err_5 = eta_i_vec(:,5) - delta_eta_vec(:,5) - eta0;
ksi_track_err_5 = ksi_i_vec(:,5) - delta_ksi_vec(:,5) - ksi0;

== matlab function sim_tase_2025_pos_ctrl/combine follower eta ksi ==
  data: ksi_track_err_vec output; ksi_track_err_1 input; ksi_track_err_2 input; ksi_track_err_3 input; ksi_track_err_4 input; ksi_track_err_5 input; eta_track_err_vec output; eta_track_err_1 input; eta_track_err_2 input; eta_track_err_3 input; eta_track_err_4 input; eta_track_err_5 input
function [ksi_track_err_vec, eta_track_err_vec]  = fcn(ksi_track_err_1, ksi_track_err_2, ksi_track_err_3, ksi_track_err_4, ksi_track_err_5, ...
                                                                                    eta_track_err_1, eta_track_err_2, eta_track_err_3, eta_track_err_4, eta_track_err_5)
%%%% 合并所有跟随者的速度/位置向量
ksi_track_err_vec = [ksi_track_err_1(:), ksi_track_err_2(:), ksi_track_err_3(:), ksi_track_err_4(:), ksi_track_err_5(:)];
eta_track_err_vec = [eta_track_err_1(:), eta_track_err_2(:), eta_track_err_3(:), eta_track_err_4(:), eta_track_err_5(:)];

== matlab function sim_tase_2025_pos_ctrl/depart Rc5 ==
  data: y output; x input
function y = fcn(x)
y = x(:,:,5);

end

== matlab function sim_tase_2025_pos_ctrl/depart Rc1 ==
  data: y output; x input
function y = fcn(x)
y = x(:,:,1);

end

== matlab function sim_tase_2025_pos_ctrl/depart Rc2 ==
  data: y output; x input
function y = fcn(x)
y = x(:,:,2);

end

== matlab function sim_tase_2025_pos_ctrl/depart Rc3 ==
  data: y output; x input
function y = fcn(x)
y = x(:,:,3);

end

== matlab function sim_tase_2025_pos_ctrl/depart Rc4 ==
  data: y output; x input
function y = fcn(x)
y = x(:,:,4);

end

== matlab function sim_tase_2025_pos_ctrl/generate translational disturbance agent 1 ==
  data: dp_aa_t input; dp_ff_t input; dp_phi_t input; dp_1 output; t input
function dp_1 = fcn(dp_aa_t, dp_ff_t, dp_phi_t, t)
%%%% 平移动力学方程中的扰动项设置
epsil_t = zeros(3, 1);

for kk = 1:5
    epsil_t = epsil_t + dp_aa_t(:, kk) .* sin( 2 * pi * dp_ff_t(:, kk) * t + dp_phi_t(:, kk) );
end

dp_1 = [ epsil_t(1) + 1.6 * sin( 0.4 * t ) + 2.0 * cos( 0.5 * t ) + 1.4 * sin( 0.7 * t ) ...
                + 4 * exp( -0.1 * t ) * sin( 0.8 * t ) + 3 / ( 1 + exp( -0.2 * ( t - 15 ) ) ); ...
                epsil_t(2) + 1.2 * sin( 0.2 * t ) + 3 * cos( 0.4 * t ) + 0.8 * sin( 0.6 * t ) ...
                + 2 * exp( -0.15 * t ) * cos( 1.2 * t ) + 3 / ( 1 + exp( -0.3 * ( t - 25 ) ) ); ...
                epsil_t(3) + 1.8 * sin( 0.2 * t ) + 1.6 * sin( 0.3 * t ) + 1.6 * cos( 0.4 * t ) ...
                + 4 * exp( -0.05 * t ) * sin( 0.5 * t + pi / 4 ) + 3 / ( 1 + exp( -0.5 * ( t - 20 ) ) ) ];

== matlab function sim_tase_2025_pos_ctrl/cal sig_ksi_diff_tilt agent 1 ==
  data: ksi_diff_tilt_vec input; sig_ksi_diff_tilt_1_2_node_1 output; ksi_diff_tilt_squ_1_2_vec input; ksi_diff_tilt_squ_gamma_1_vec input; ksi_diff_tilt_squ_gamma_2_2_vec input; sig_ksi_diff_tilt_gamma_1_node_1 output; sig_ksi_diff_tilt_gamma_2_2_node_1 output
function [sig_ksi_diff_tilt_1_2_node_1, sig_ksi_diff_tilt_gamma_1_node_1, sig_ksi_diff_tilt_gamma_2_2_node_1] = fcn(ksi_diff_tilt_vec, ksi_diff_tilt_squ_1_2_vec, ...
                                                                                                                                                                                                                    ksi_diff_tilt_squ_gamma_1_vec, ...
                                                                                                                                                                                                                    ksi_diff_tilt_squ_gamma_2_2_vec)
%%%% 计算高阶滑模微分器中所使用的sig函数
iiuav = 1;
sig_ksi_diff_tilt_1_2_node_1 = ksi_diff_tilt_squ_1_2_vec(:,iiuav) .* sign( ksi_diff_tilt_vec(:,iiuav) );
sig_ksi_diff_tilt_gamma_1_node_1 = ksi_diff_tilt_squ_gamma_1_vec(:,iiuav) .* sign( ksi_diff_tilt_vec(:,iiuav) );
sig_ksi_diff_tilt_gamma_2_2_node_1 = ksi_diff_tilt_squ_gamma_2_2_vec(:,iiuav) .* sign( ksi_diff_tilt_vec(:,iiuav) );

== matlab function sim_tase_2025_pos_ctrl/combine ksi_diff_tilt_squ_1_2 ==
  data: ksi_diff_tilt_squ_1_2_node_1 input; ksi_diff_tilt_squ_1_2_vec output; ksi_diff_tilt_squ_1_2_node_2 input; ksi_diff_tilt_squ_1_2_node_3 input; ksi_diff_tilt_squ_1_2_node_4 input; ksi_diff_tilt_squ_1_2_node_5 input
function ksi_diff_tilt_squ_1_2_vec = fcn(ksi_diff_tilt_squ_1_2_node_1, ksi_diff_tilt_squ_1_2_node_2, ...
                                                                        ksi_diff_tilt_squ_1_2_node_3, ksi_diff_tilt_squ_1_2_node_4, ...
                                                                        ksi_diff_tilt_squ_1_2_node_5)
%%%% 合并绝对值幂次项
ksi_diff_tilt_squ_1_2_vec = zeros(3,5);
ksi_diff_tilt_squ_1_2_vec(:,1) = ksi_diff_tilt_squ_1_2_node_1(:);
ksi_diff_tilt_squ_1_2_vec(:,2) = ksi_diff_tilt_squ_1_2_node_2(:);
ksi_diff_tilt_squ_1_2_vec(:,3) = ksi_diff_tilt_squ_1_2_node_3(:);
ksi_diff_tilt_squ_1_2_vec(:,4) = ksi_diff_tilt_squ_1_2_node_4(:);
ksi_diff_tilt_squ_1_2_vec(:,5) = ksi_diff_tilt_squ_1_2_node_5(:);

== matlab function sim_tase_2025_pos_ctrl/combine ksi_diff_tilt_squ_gamma_1 ==
  data: ksi_diff_tilt_squ_gamma_1_node_1 input; ksi_diff_tilt_squ_gamma_1_vec output; ksi_diff_tilt_squ_gamma_1_node_2 input; ksi_diff_tilt_squ_gamma_1_node_3 input; ksi_diff_tilt_squ_gamma_1_node_4 input; ksi_diff_tilt_squ_gamma_1_node_5 input
function ksi_diff_tilt_squ_gamma_1_vec = fcn(ksi_diff_tilt_squ_gamma_1_node_1, ksi_diff_tilt_squ_gamma_1_node_2, ...
                                                                                    ksi_diff_tilt_squ_gamma_1_node_3, ksi_diff_tilt_squ_gamma_1_node_4, ...
                                                                                    ksi_diff_tilt_squ_gamma_1_node_5)
%%%% 合并绝对值幂次项
ksi_diff_tilt_squ_gamma_1_vec = zeros(3,5);
ksi_diff_tilt_squ_gamma_1_vec(:,1) = ksi_diff_tilt_squ_gamma_1_node_1(:);
ksi_diff_tilt_squ_gamma_1_vec(:,2) = ksi_diff_tilt_squ_gamma_1_node_2(:);
ksi_diff_tilt_squ_gamma_1_vec(:,3) = ksi_diff_tilt_squ_gamma_1_node_3(:);
ksi_diff_tilt_squ_gamma_1_vec(:,4) = ksi_diff_tilt_squ_gamma_1_node_4(:);
ksi_diff_tilt_squ_gamma_1_vec(:,5) = ksi_diff_tilt_squ_gamma_1_node_5(:);

== matlab function sim_tase_2025_pos_ctrl/combine ksi_diff_tilt_squ_gamma_2_2 ==
  data: ksi_diff_tilt_squ_gamma_2_2_node_1 input; ksi_diff_tilt_squ_gamma_2_2_vec output; ksi_diff_tilt_squ_gamma_2_2_node_2 input; ksi_diff_tilt_squ_gamma_2_2_node_3 input; ksi_diff_tilt_squ_gamma_2_2_node_4 input; ksi_diff_tilt_squ_gamma_2_2_node_5 input
function ksi_diff_tilt_squ_gamma_2_2_vec = fcn(ksi_diff_tilt_squ_gamma_2_2_node_1, ksi_diff_tilt_squ_gamma_2_2_node_2, ...
                                                                                        ksi_diff_tilt_squ_gamma_2_2_node_3, ksi_diff_tilt_squ_gamma_2_2_node_4, ...
                                                                                        ksi_diff_tilt_squ_gamma_2_2_node_5)
%%%% 合并绝对值幂次项
ksi_diff_tilt_squ_gamma_2_2_vec = zeros(3,5);
ksi_diff_tilt_squ_gamma_2_2_vec(:,1) = ksi_diff_tilt_squ_gamma_2_2_node_1(:);
ksi_diff_tilt_squ_gamma_2_2_vec(:,2) = ksi_diff_tilt_squ_gamma_2_2_node_2(:);
ksi_diff_tilt_squ_gamma_2_2_vec(:,3) = ksi_diff_tilt_squ_gamma_2_2_node_3(:);
ksi_diff_tilt_squ_gamma_2_2_vec(:,4) = ksi_diff_tilt_squ_gamma_2_2_node_4(:);
ksi_diff_tilt_squ_gamma_2_2_vec(:,5) = ksi_diff_tilt_squ_gamma_2_2_node_5(:);

== matlab function sim_tase_2025_pos_ctrl/cal abs 2 ==
  data: x input; y output
function y = fcn(x)
y = abs(x(:));

== matlab function sim_tase_2025_pos_ctrl/cal abs 3 ==
  data: x input; y output
function y = fcn(x)
y = abs(x(:));

== matlab function sim_tase_2025_pos_ctrl/cal abs 4 ==
  data: x input; y output
function y = fcn(x)
y = abs(x(:));

== matlab function sim_tase_2025_pos_ctrl/cal sig_ksi_diff_tilt agent 2 ==
  data: ksi_diff_tilt_vec input; sig_ksi_diff_tilt_1_2_node_2 output; ksi_diff_tilt_squ_1_2_vec input; ksi_diff_tilt_squ_gamma_1_vec input; ksi_diff_tilt_squ_gamma_2_2_vec input; sig_ksi_diff_tilt_gamma_1_node_2 output; sig_ksi_diff_tilt_gamma_2_2_node_2 output
function [sig_ksi_diff_tilt_1_2_node_2, sig_ksi_diff_tilt_gamma_1_node_2, sig_ksi_diff_tilt_gamma_2_2_node_2] = fcn(ksi_diff_tilt_vec, ksi_diff_tilt_squ_1_2_vec, ...
                                                                                                                                                                                                                    ksi_diff_tilt_squ_gamma_1_vec, ...
                                                                                                                                                                                                                    ksi_diff_tilt_squ_gamma_2_2_vec)
%%%% 计算高阶滑模微分器中所使用的sig函数
iiuav = 2;
sig_ksi_diff_tilt_1_2_node_2 = ksi_diff_tilt_squ_1_2_vec(:,iiuav) .* sign( ksi_diff_tilt_vec(:,iiuav) );
sig_ksi_diff_tilt_gamma_1_node_2 = ksi_diff_tilt_squ_gamma_1_vec(:,iiuav) .* sign( ksi_diff_tilt_vec(:,iiuav) );
sig_ksi_diff_tilt_gamma_2_2_node_2 = ksi_diff_tilt_squ_gamma_2_2_vec(:,iiuav) .* sign( ksi_diff_tilt_vec(:,iiuav) );

== matlab function sim_tase_2025_pos_ctrl/choose ksi_diff_tilt 3 ==
  data: x input; y output
function y = fcn(x)
iiuav = 2;
y = x(:,iiuav);

== matlab function sim_tase_2025_pos_ctrl/choose ksi_diff_tilt 4 ==
  data: x input; y output
function y = fcn(x)
iiuav = 2;
y = x(:,iiuav);

== matlab function sim_tase_2025_pos_ctrl/choose ksi_diff_tilt1 ==
  data: x input; y output
function y = fcn(x)
iiuav = 2;
y = x(:,iiuav);

== matlab function sim_tase_2025_pos_ctrl/generate translational disturbance agent 2 ==
  data: dp_aa_t input; dp_ff_t input; dp_phi_t input; dp_2 output; t input
function dp_2 = fcn(dp_aa_t, dp_ff_t, dp_phi_t, t)
%%%% 平移动力学方程中的扰动项设置
epsil_t = zeros(3, 1);

for kk = 1:5
    epsil_t = epsil_t + dp_aa_t(:, kk) .* sin( 2 * pi * dp_ff_t(:, kk) * t + dp_phi_t(:, kk) );
end

dp_2 = [ epsil_t(1) + 1.6 * sin( 0.2 * t ) + 2.0 * cos( 0.3 * t ) + 1.4 * sin( 0.5 * t ) ...
                + 4 * exp( -0.1 * t ) * sin( 0.5 * t ) + 3 / ( 1 + exp( -0.2 * ( t - 15 ) ) ); ...
                epsil_t(2) + 1.2 * sin( 0.1 * t ) + 3 * cos( 0.2 * t ) + 0.8 * sin( 0.4 * t ) ...
                + 2 * exp( -0.15 * t ) * cos( 0.6 * t ) + 3 / ( 1 + exp( -0.3 * ( t - 25 ) ) ); ...
                epsil_t(3) + 1.8 * sin( 0.1 * t ) + 1.6 * sin( 0.2 * t ) + 1.6 * cos( 0.3 * t ) ...
                + 4 * exp( -0.05 * t ) * sin( 0.4 * t + pi / 4 ) + 3 / ( 1 + exp( -0.5 * ( t - 20 ) ) ) ];

== matlab function sim_tase_2025_pos_ctrl/trans to column2 ==
  data: x input; y output
function y = fcn(x)
y = x(:);

== matlab function sim_tase_2025_pos_ctrl/trans to column3 ==
  data: x input; y output
function y = fcn(x)
y = x(:);

== matlab function sim_tase_2025_pos_ctrl/trans to column4 ==
  data: x input; y output
function y = fcn(x)
y = x(:);

== matlab function sim_tase_2025_pos_ctrl/cal abs 5 ==
  data: x input; y output
function y = fcn(x)
y = abs(x(:));

== matlab function sim_tase_2025_pos_ctrl/cal abs 6 ==
  data: x input; y output
function y = fcn(x)
y = abs(x(:));

== matlab function sim_tase_2025_pos_ctrl/cal abs 7 ==
  data: x input; y output
function y = fcn(x)
y = abs(x(:));

== matlab function sim_tase_2025_pos_ctrl/cal sig_ksi_diff_tilt agent 3 ==
  data: ksi_diff_tilt_vec input; sig_ksi_diff_tilt_1_2_node_3 output; ksi_diff_tilt_squ_1_2_vec input; ksi_diff_tilt_squ_gamma_1_vec input; ksi_diff_tilt_squ_gamma_2_2_vec input; sig_ksi_diff_tilt_gamma_1_node_3 output; sig_ksi_diff_tilt_gamma_2_2_node_3 output
function [sig_ksi_diff_tilt_1_2_node_3, sig_ksi_diff_tilt_gamma_1_node_3, sig_ksi_diff_tilt_gamma_2_2_node_3] = fcn(ksi_diff_tilt_vec, ksi_diff_tilt_squ_1_2_vec, ...
                                                                                                                                                                                                                    ksi_diff_tilt_squ_gamma_1_vec, ...
                                                                                                                                                                                                                    ksi_diff_tilt_squ_gamma_2_2_vec)
%%%% 计算高阶滑模微分器中所使用的sig函数
iiuav = 3;
sig_ksi_diff_tilt_1_2_node_3 = ksi_diff_tilt_squ_1_2_vec(:,iiuav) .* sign( ksi_diff_tilt_vec(:,iiuav) );
sig_ksi_diff_tilt_gamma_1_node_3 = ksi_diff_tilt_squ_gamma_1_vec(:,iiuav) .* sign( ksi_diff_tilt_vec(:,iiuav) );
sig_ksi_diff_tilt_gamma_2_2_node_3 = ksi_diff_tilt_squ_gamma_2_2_vec(:,iiuav) .* sign( ksi_diff_tilt_vec(:,iiuav) );

== matlab function sim_tase_2025_pos_ctrl/choose ksi_diff_tilt 5 ==
  data: x input; y output
function y = fcn(x)
iiuav = 3;
y = x(:,iiuav);

== matlab function sim_tase_2025_pos_ctrl/choose ksi_diff_tilt 6 ==
  data: x input; y output
function y = fcn(x)
iiuav = 3;
y = x(:,iiuav);

== matlab function sim_tase_2025_pos_ctrl/choose ksi_diff_tilt2 ==
  data: x input; y output
function y = fcn(x)
iiuav = 3;
y = x(:,iiuav);

== matlab function sim_tase_2025_pos_ctrl/trans to column5 ==
  data: x input; y output
function y = fcn(x)
y = x(:);

== matlab function sim_tase_2025_pos_ctrl/trans to column6 ==
  data: x input; y output
function y = fcn(x)
y = x(:);

== matlab function sim_tase_2025_pos_ctrl/trans to column7 ==
  data: x input; y output
function y = fcn(x)
y = x(:);

== matlab function sim_tase_2025_pos_ctrl/cal abs 10 ==
  data: x input; y output
function y = fcn(x)
y = abs(x(:));

== matlab function sim_tase_2025_pos_ctrl/generate translational disturbance agent 3 ==
  data: dp_aa_t input; dp_ff_t input; dp_phi_t input; dp_3 output; t input
function dp_3 = fcn(dp_aa_t, dp_ff_t, dp_phi_t, t)
%%%% 平移动力学方程中的扰动项设置
epsil_t = zeros(3, 1);

for kk = 1:5
    epsil_t = epsil_t + dp_aa_t(:, kk) .* sin( 2 * pi * dp_ff_t(:, kk) * t + dp_phi_t(:, kk) );
end

dp_3 = [ epsil_t(1) + 1.6 * sin( 0.2 * t ) + 2.0 * cos( 0.3 * t ) + 1.4 * sin( 0.5 * t ) ...
                + 4 * exp( -0.1 * t ) * sin( 0.5 * t ) + 3 / ( 1 + exp( -0.2 * ( t - 15 ) ) ); ...
                epsil_t(2) + 1.2 * sin( 0.1 * t ) + 3 * cos( 0.2 * t ) + 0.8 * sin( 0.4 * t ) ...
                + 2 * exp( -0.15 * t ) * cos( 0.6 * t ) + 3 / ( 1 + exp( -0.3 * ( t - 25 ) ) ); ...
                epsil_t(3) + 1.8 * sin( 0.1 * t ) + 1.6 * sin( 0.2 * t ) + 1.6 * cos( 0.3 * t ) ...
                + 4 * exp( -0.05 * t ) * sin( 0.4 * t + pi / 4 ) + 3 / ( 1 + exp( -0.5 * ( t - 20 ) ) ) ];

== matlab function sim_tase_2025_pos_ctrl/cal abs 8 ==
  data: x input; y output
function y = fcn(x)
y = abs(x(:));

== matlab function sim_tase_2025_pos_ctrl/cal abs 9 ==
  data: x input; y output
function y = fcn(x)
y = abs(x(:));

== matlab function sim_tase_2025_pos_ctrl/cal sig_ksi_diff_tilt agent 4 ==
  data: ksi_diff_tilt_vec input; sig_ksi_diff_tilt_1_2_node_4 output; ksi_diff_tilt_squ_1_2_vec input; ksi_diff_tilt_squ_gamma_1_vec input; ksi_diff_tilt_squ_gamma_2_2_vec input; sig_ksi_diff_tilt_gamma_1_node_4 output; sig_ksi_diff_tilt_gamma_2_2_node_4 output
function [sig_ksi_diff_tilt_1_2_node_4, sig_ksi_diff_tilt_gamma_1_node_4, sig_ksi_diff_tilt_gamma_2_2_node_4] = fcn(ksi_diff_tilt_vec, ksi_diff_tilt_squ_1_2_vec, ...
                                                                                                                                                                                                                    ksi_diff_tilt_squ_gamma_1_vec, ...
                                                                                                                                                                                                                    ksi_diff_tilt_squ_gamma_2_2_vec)
%%%% 计算高阶滑模微分器中所使用的sig函数
iiuav = 4;
sig_ksi_diff_tilt_1_2_node_4 = ksi_diff_tilt_squ_1_2_vec(:,iiuav) .* sign( ksi_diff_tilt_vec(:,iiuav) );
sig_ksi_diff_tilt_gamma_1_node_4 = ksi_diff_tilt_squ_gamma_1_vec(:,iiuav) .* sign( ksi_diff_tilt_vec(:,iiuav) );
sig_ksi_diff_tilt_gamma_2_2_node_4 = ksi_diff_tilt_squ_gamma_2_2_vec(:,iiuav) .* sign( ksi_diff_tilt_vec(:,iiuav) );

== matlab function sim_tase_2025_pos_ctrl/choose ksi_diff_tilt 7 ==
  data: x input; y output
function y = fcn(x)
iiuav = 4;
y = x(:,iiuav);

== matlab function sim_tase_2025_pos_ctrl/choose ksi_diff_tilt 8 ==
  data: x input; y output
function y = fcn(x)
iiuav = 4;
y = x(:,iiuav);

== matlab function sim_tase_2025_pos_ctrl/choose ksi_diff_tilt3 ==
  data: x input; y output
function y = fcn(x)
iiuav = 4;
y = x(:,iiuav);

== matlab function sim_tase_2025_pos_ctrl/trans to column10 ==
  data: x input; y output
function y = fcn(x)
y = x(:);

== matlab function sim_tase_2025_pos_ctrl/trans to column8 ==
  data: x input; y output
function y = fcn(x)
y = x(:);

== matlab function sim_tase_2025_pos_ctrl/trans to column9 ==
  data: x input; y output
function y = fcn(x)
y = x(:);

== matlab function sim_tase_2025_pos_ctrl/cal abs 11 ==
  data: x input; y output
function y = fcn(x)
y = abs(x(:));

== matlab function sim_tase_2025_pos_ctrl/cal abs 12 ==
  data: x input; y output
function y = fcn(x)
y = abs(x(:));

== matlab function sim_tase_2025_pos_ctrl/cal abs 13 ==
  data: x input; y output
function y = fcn(x)
y = abs(x(:));

== matlab function sim_tase_2025_pos_ctrl/cal sig_ksi_diff_tilt agent 5 ==
  data: ksi_diff_tilt_vec input; sig_ksi_diff_tilt_1_2_node_5 output; ksi_diff_tilt_squ_1_2_vec input; ksi_diff_tilt_squ_gamma_1_vec input; ksi_diff_tilt_squ_gamma_2_2_vec input; sig_ksi_diff_tilt_gamma_1_node_5 output; sig_ksi_diff_tilt_gamma_2_2_node_5 output
function [sig_ksi_diff_tilt_1_2_node_5, sig_ksi_diff_tilt_gamma_1_node_5, sig_ksi_diff_tilt_gamma_2_2_node_5] = fcn(ksi_diff_tilt_vec, ksi_diff_tilt_squ_1_2_vec, ...
                                                                                                                                                                                                                    ksi_diff_tilt_squ_gamma_1_vec, ...
                                                                                                                                                                                                                    ksi_diff_tilt_squ_gamma_2_2_vec)
%%%% 计算高阶滑模微分器中所使用的sig函数
iiuav = 5;
sig_ksi_diff_tilt_1_2_node_5 = ksi_diff_tilt_squ_1_2_vec(:,iiuav) .* sign( ksi_diff_tilt_vec(:,iiuav) );
sig_ksi_diff_tilt_gamma_1_node_5 = ksi_diff_tilt_squ_gamma_1_vec(:,iiuav) .* sign( ksi_diff_tilt_vec(:,iiuav) );
sig_ksi_diff_tilt_gamma_2_2_node_5 = ksi_diff_tilt_squ_gamma_2_2_vec(:,iiuav) .* sign( ksi_diff_tilt_vec(:,iiuav) );

== matlab function sim_tase_2025_pos_ctrl/generate translational disturbance agent 4 ==
  data: dp_aa_t input; dp_ff_t input; dp_phi_t input; dp_4 output; t input
function dp_4 = fcn(dp_aa_t, dp_ff_t, dp_phi_t, t)
%%%% 平移动力学方程中的扰动项设置
epsil_t = zeros(3, 1);

for kk = 1:5
    epsil_t = epsil_t + dp_aa_t(:, kk) .* sin( 2 * pi * dp_ff_t(:, kk) * t + dp_phi_t(:, kk) );
end

dp_4 = [ epsil_t(1) + 1.6 * sin( 0.2 * t ) + 2.0 * cos( 0.3 * t ) + 1.4 * sin( 0.5 * t ) ...
                + 4 * exp( -0.1 * t ) * sin( 0.5 * t ) + 3 / ( 1 + exp( -0.2 * ( t - 15 ) ) ); ...
                epsil_t(2) + 1.2 * sin( 0.1 * t ) + 3 * cos( 0.2 * t ) + 0.8 * sin( 0.4 * t ) ...
                + 2 * exp( -0.15 * t ) * cos( 0.6 * t ) + 3 / ( 1 + exp( -0.3 * ( t - 25 ) ) ); ...
                epsil_t(3) + 1.8 * sin( 0.1 * t ) + 1.6 * sin( 0.2 * t ) + 1.6 * cos( 0.3 * t ) ...
                + 4 * exp( -0.05 * t ) * sin( 0.4 * t + pi / 4 ) + 3 / ( 1 + exp( -0.5 * ( t - 20 ) ) ) ];

== matlab function sim_tase_2025_pos_ctrl/choose ksi_diff_tilt 10 ==
  data: x input; y output
function y = fcn(x)
iiuav = 5;
y = x(:,iiuav);

== matlab function sim_tase_2025_pos_ctrl/choose ksi_diff_tilt 9 ==
  data: x input; y output
function y = fcn(x)
iiuav = 5;
y = x(:,iiuav);

== matlab function sim_tase_2025_pos_ctrl/choose ksi_diff_tilt4 ==
  data: x input; y output
function y = fcn(x)
iiuav = 5;
y = x(:,iiuav);

== matlab function sim_tase_2025_pos_ctrl/trans to column11 ==
  data: x input; y output
function y = fcn(x)
y = x(:);

== matlab function sim_tase_2025_pos_ctrl/trans to column12 ==
  data: x input; y output
function y = fcn(x)
y = x(:);

== matlab function sim_tase_2025_pos_ctrl/trans to column13 ==
  data: x input; y output
function y = fcn(x)
y = x(:);

== matlab function sim_tase_2025_pos_ctrl/combine sig_ksi_diff_tilt_1_2 ==
  data: sig_ksi_diff_tilt_1_2_node_1 input; sig_ksi_diff_tilt_1_2_vec output; sig_ksi_diff_tilt_1_2_node_2 input; sig_ksi_diff_tilt_1_2_node_3 input; sig_ksi_diff_tilt_1_2_node_4 input; sig_ksi_diff_tilt_1_2_node_5 input
function sig_ksi_diff_tilt_1_2_vec = fcn(sig_ksi_diff_tilt_1_2_node_1, sig_ksi_diff_tilt_1_2_node_2, ...
                                                                        sig_ksi_diff_tilt_1_2_node_3, sig_ksi_diff_tilt_1_2_node_4, ...
                                                                        sig_ksi_diff_tilt_1_2_node_5)
%%%% 合并绝对值幂次项
sig_ksi_diff_tilt_1_2_vec = zeros(3,5);
sig_ksi_diff_tilt_1_2_vec(:,1) = sig_ksi_diff_tilt_1_2_node_1(:);
sig_ksi_diff_tilt_1_2_vec(:,2) = sig_ksi_diff_tilt_1_2_node_2(:);
sig_ksi_diff_tilt_1_2_vec(:,3) = sig_ksi_diff_tilt_1_2_node_3(:);
sig_ksi_diff_tilt_1_2_vec(:,4) = sig_ksi_diff_tilt_1_2_node_4(:);
sig_ksi_diff_tilt_1_2_vec(:,5) = sig_ksi_diff_tilt_1_2_node_5(:);

== matlab function sim_tase_2025_pos_ctrl/combine sig_ksi_diff_tilt_gamma_1 ==
  data: sig_ksi_diff_tilt_gamma_1_node_1 input; sig_ksi_diff_tilt_gamma_1_vec output; sig_ksi_diff_tilt_gamma_1_node_2 input; sig_ksi_diff_tilt_gamma_1_node_3 input; sig_ksi_diff_tilt_gamma_1_node_4 input; sig_ksi_diff_tilt_gamma_1_node_5 input
function sig_ksi_diff_tilt_gamma_1_vec = fcn(sig_ksi_diff_tilt_gamma_1_node_1, sig_ksi_diff_tilt_gamma_1_node_2, ...
                                                                                    sig_ksi_diff_tilt_gamma_1_node_3, sig_ksi_diff_tilt_gamma_1_node_4, ...
                                                                                    sig_ksi_diff_tilt_gamma_1_node_5)
%%%% 合并绝对值幂次项
sig_ksi_diff_tilt_gamma_1_vec = zeros(3,5);
sig_ksi_diff_tilt_gamma_1_vec(:,1) = sig_ksi_diff_tilt_gamma_1_node_1(:);
sig_ksi_diff_tilt_gamma_1_vec(:,2) = sig_ksi_diff_tilt_gamma_1_node_2(:);
sig_ksi_diff_tilt_gamma_1_vec(:,3) = sig_ksi_diff_tilt_gamma_1_node_3(:);
sig_ksi_diff_tilt_gamma_1_vec(:,4) = sig_ksi_diff_tilt_gamma_1_node_4(:);
sig_ksi_diff_tilt_gamma_1_vec(:,5) = sig_ksi_diff_tilt_gamma_1_node_5(:);
